simulink model "CPS_PowerSync_System"  (R2024a)
settings: Solver=FixedStepAuto  StartTime=0.0  StopTime=50  FixedStep=0.1  RelTol=1e-3
model workspace (MAT data in the model file):
  SoC = Simulink.Signal
  SoC.DataType = 'double'
  SoC.Dimensions = -1
  SoC.DimensionsMode = 'auto'
  SoC.Complexity = 'auto'
  SoC.SampleTime = -1
  SoC.SamplingMode = 'auto'
undefined symbols (not defined in the file or in its folder): m, v_CP1, v_CP2, v_CP3, w_CP1, w_CP2, w_CP3
(part 1 of 3)
settings Model: SimulationMode=accelerator  SnapshotBufferSize=100  SnapshotInterval=1  Creator=rober  LastModifiedBy=gabri
settings SolverCC: ConcurrentTasks=on  AutoInsertRateTranBlk=on
settings DebuggingCC: BusObjectLabelMismatch=none  UnderSpecifiedDimensionMsg=warning

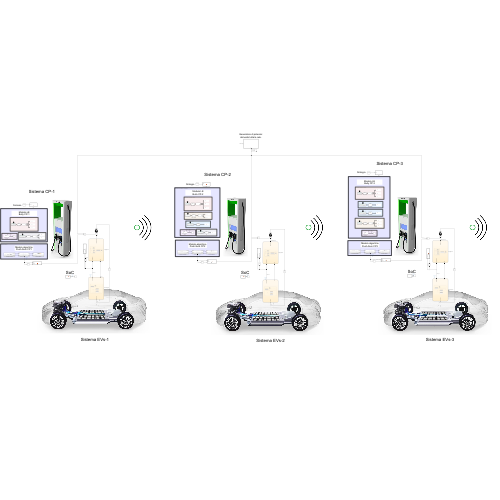
[thumbnail: Simulink's stored preview of the top-level diagram]
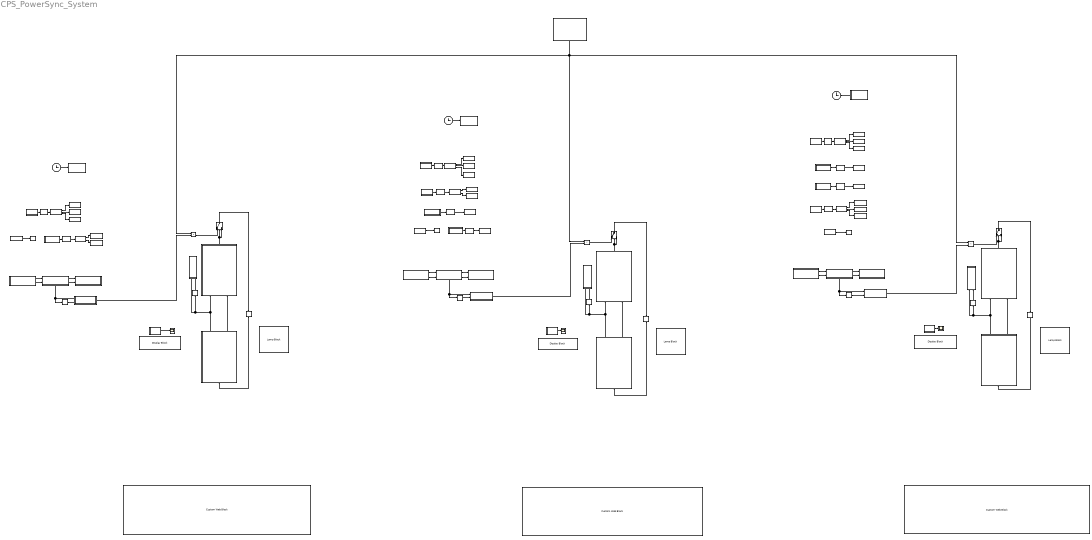
== system CPS_PowerSync_System ==
  note: Sistema EVs-3
  note: Answer module for LE
  note: Send Module
  note: Receive module
  note: Charging point 1 | UID 1 | LE module 1
  note: Charging Point 3 | UID 3 | LE module 3
  note: Charging point 2 | UID 2 | LE module 2
  note: Receive module
  note: Send Module
  note: Receive module
  note: Leader dead notification module
  note: Push-sum module 3
  note: Push-sum module 1
  note: Push-sum module 2
  note: Orologio
  note: Modulo LE
      | Bully CP-1
  note: Modulo algoritmo
      | Push-Sum CP1
  note: Modulo algoritmo
      | Push-Sum CP2
  note: Modulo algoritmo
      | Push-Sum CP3
  note: Answer module for LE
  note: Election notification module
  note: Generatore di potenza: alimenta tutta la rete.
  note: Sistema CP-2
  note: Sistema CP-3
  note: Sistema CP-1
  note: Sistema EVs-1
  note: Sistema EVs-2
  note: SoC
  note: Modulo LE
      | Bully CP-2
  note: Modulo LE
      | Bully CP-3
  note: Leader dead notification module
  note: Election notification module
  note: Orologio
  note: Orologio
  note: Leader dead notification module
  note: Answer module for LE
  note: SoC
  note: SoC
  CP 1 : EntityGenerator  InputPortMessageModes=m  OutputPortMessageModes=m  GenerationMethod=Event-based  TimeSource=Signal port  Period=3  AttributeName=UID  EntityType=Structured  EntityTypeName=Entity
      settings: InputPortMap=u0
  CP 2 : EntityGenerator  InputPortMessageModes=m  OutputPortMessageModes=m  GenerationMethod=Event-based  TimeSource=Signal port  Period=3  AttributeName=UID  AttributeInitialValue=2  EntityType=Structured  EntityTypeName=Entity
      settings: InputPortMap=u0
  CP1 : MATLAB Function  TreatAsAtomicUnit=on
  CP2 : MATLAB Function  TreatAsAtomicUnit=on
  CP3 : MATLAB Function  TreatAsAtomicUnit=on
  ChargingPoint1 : Stateflow chart  TreatAsAtomicUnit=on
  ChargingPoint2 : Stateflow chart  TreatAsAtomicUnit=on
  ChargingPoint3 : Stateflow chart  TreatAsAtomicUnit=on
  Clock1 : Clock
  Clock2 : Clock
  Clock3 : Clock
  Delay{,1..8} (9 alike) : Delay  DelayLength=1  InitialCondition=0  SampleTime=0.1
  Display : DisplayBlock  LabelPosition=Hide  Transparency=1
  Display2 : DisplayBlock  LabelPosition=Hide  Transparency=1
  Display3 : DisplayBlock  LabelPosition=Hide  Transparency=1
  ElecritcVehicles1 : Stateflow chart  TreatAsAtomicUnit=on
  ElecritcVehicles2 : Stateflow chart  TreatAsAtomicUnit=on
  ElecritcVehicles3 : Stateflow chart  TreatAsAtomicUnit=on
  Entity Multicast{,6,8,11,13..14,16} (7 alike) : EntityMulticast  Tag=B  InputPortMessageModes=m  MulticastTag=B
  Entity Multicast{1,4,7,9..10,18..19} (7 alike) : EntityMulticast  Tag=A  InputPortMessageModes=m
  Entity Multicast{2..3,5,12,15,17} (6 alike) : EntityMulticast  Tag=C  InputPortMessageModes=m  MulticastTag=C
  Entity Replicator{,1,4..5} (4 alike) : EntityReplicator  InputPortMessageModes=m  OutputPortMessageModes=m,m,m  NumberReplicas=2
      settings: OutputPortMap=o0,o1,o2
  Entity Replicator2 : EntityReplicator  InputPortMessageModes=m  OutputPortMessageModes=m,m
  Entity Replicator3 : EntityReplicator  InputPortMessageModes=m  OutputPortMessageModes=m,m
  Entity Terminator : EntityTerminator  InputPortMessageModes=m  EntryAction=|
      | coder.extrinsic('evalin');
      | coder.extrinsic('assignin');
      | 
      | check_variables('v_CP1');
      | 
      | clock = 0;
      | clock = evalin('base', 'clock_CP1');
      | 
      | pr_actual = 0;
      | pr_actual = evalin('base', 'double(pr_actual_CP1)');
      | 
      | if pr_actual == 0
      |     assignin('base', 'v_CP1', 0); % Non sono leader
      | end
      | 
      | % Caso in cui ricevo un UID maggiore del mio
      | if entity.UID > 1
      |     assignin('base', 'flg_response_CP1', 1);
      |     assignin('base', 'v_CP1', 0); % Non sono leader
      |     disp('CP1 received a UID greater than its own, so it knows that it will not be the leader.')
      | end
      | 
      | 
      | % Caso in cui ricevo messaggio di elezione avvenuta e sono connesso
      | if entity.UID == -2 && pr_actual == 1
      |     
      |     % Elezione avvenuta
      |     % Tutti e tre questi flag sono necessari al corretto funzionamento dell'algoritmo push-sum
      |     assignin('base', 'flg_elected_CP1', 1);
      |     assignin('base', 'flg_first_instant_v_CP1', 1);
      |     assignin('base', 'flg_first_instant_w_CP1', 1);
      | 
      |     assignin('base', 'flg_send_CP1', 0);
      |     
      |     disp('CP1 is active and has learned that the leader has been elected (received -2).')
      | 
      | end
      | 
      | 
      | % Ricevo notifica morte leader
      | if entity.UID == -1
      |     
      |     disp('CP1 heard that the leader died (received -1)')
      |     
      |     % Reset del valore e del peso
      |     assignin('base', 'v_CP1', 0);
      |     assignin('base', 'w_CP1', 0);
      |     
      |     % Il leader deve essere rieletto, quindi flag_elected viene riportato a zero
      |     assignin('base', 'flg_elected_CP1', 0);
      |     
      |     % Il nodo si propone come leader e, nel caso in cui riceverà
      |     % una risposta, questo flag sarà impostato = 1
      |     assignin('base', 'flg_response_CP1', 0);
      |     
      |     % Flag necessari a far ripartire l'algoritmo push-sum correttamente
      |     assignin('base', 'flg_dead_v_CP1', 1);
      |     assignin('base', 'flg_dead_w_CP1', 1);
      |     assignin('base', 'flg_reset_v_CP1', 1);
      |     assignin('base', 'flg_reset_w_CP1', 1);
      | 
      |     if pr_actual == 1
      |         
      |         disp('CP1 sent its candidacy.')
      | 
      |         % Il nodo si propone come leader inviando il messaggio
      |         get_event_CP1();
      |         assignin('base', 'flg_send_CP1', 1);
      |         
      |         % Stacco il tempo (tempo di invio del messaggio)
      |         assignin('base', 't_send_CP1', clock);
      |         
      |     end
      | 
      | end
  Entity Terminator1 : EntityTerminator  InputPortMessageModes=m  EntryAction=|
      | coder.extrinsic('evalin');
      | coder.extrinsic('assignin');
      | 
      | check_variables('v_CP2');
      | 
      | clock = 0;
      | clock = evalin('base', 'clock_CP2');
      | 
      | pr_actual = 0;
      | pr_actual = evalin('base', 'double(pr_actual_CP2)');
      | 
      | t_send = 0;
      | t_send = evalin('base', 't_send_CP2');
      | 
      | if pr_actual == 0
      |     assignin('base', 'v_CP2', 0); % Non sono leader
      | end
      | 
      | 
      | % Caso in cui ricevo un UID maggiore del mio
      | if entity.UID > 2
      |     assignin('base', 'flg_response_CP2', 1);
      |     assignin('base', 'v_CP2', 0); % Non sono leader
      |     disp('CP2 received a UID greater than its own, so it knows that it will not be the leader.')
      | end
      | 
      | 
      | % Se sei connesso e ti contatta un nodo con UID più piccolo rispondi
      | if entity.UID < 2 && entity.UID > 0 && pr_actual == 1
      |     
      |     response_2_to_1();
      |     
      |     assignin('base', 'flg_send_CP2', 1);
      |     
      |     if (clock - t_send) > 1
      |         assignin('base', 't_send_CP2', clock);
      |     end
      |     
      |     disp('CP2 received UID = 1, so it responds to CP1.')
      |     
      | end
      | 
      | % Caso in cui ricevo messaggio di elezione avvenuta e sono connesso
      | if entity.UID == -2 && pr_actual == 1
      |     
      |     % Elezione avvenuta
      |     % Tutti e tre questi flag sono necessari al corretto funzionamento dell'algoritmo push-sum
      |     assignin('base', 'flg_elected_CP2', 1);
      |     assignin('base', 'flg_first_instant_v_CP2', 1);
      |     assignin('base', 'flg_first_instant_w_CP2', 1);
      | 
      |     assignin('base', 'flg_send_CP2', 0);
      |     
      |     disp('CP2 is active and has learned that the leader has been elected (received -2).')
      | 
      | end
      | 
      | 
      | % Ricevo notifica morte leader
      | if entity.UID == -1
      |     
      |     disp('CP2 heard that the leader died (received -1)')
      |     
      |     % Reset del valore e del peso
      |     assignin('base', 'v_CP2', 0);
      |     assignin('base', 'w_CP2', 0);
      |     
      |     % Il leader deve essere rieletto, quindi flag_elected viene riportato a zero
      |     assignin('base', 'flg_elected_CP2', 0);
      |     
      |     % Il nodo si propone come leader e, nel caso in cui riceverà
      |     % una risposta, questo flag sarà impostato = 1
      |     assignin('base', 'flg_response_CP2', 0);
      |     
      |     % Flag necessari a far ripartire l'algoritmo push-sum correttamente
      |     assignin('base', 'flg_dead_v_CP2', 1);
      |     assignin('base', 'flg_dead_w_CP2', 1);
      |     assignin('base', 'flg_reset_v_CP2', 1);
      |     assignin('base', 'flg_reset_w_CP2', 1);
      | 
      |     if pr_actual == 1
      |         
      |         disp('CP2 sent its candidacy.')
      | 
      |         % Il nodo si propone come leader inviando il messaggio
      |         get_event_CP2();
      |         assignin('base', 'flg_send_CP2', 1);
      |         
      |         % Stacco il tempo (tempo di invio del messaggio)
      |         assignin('base', 't_send_CP2', clock);
      |         
      |     end
      | 
      | end
  Entity Terminator2 : EntityTerminator  InputPortMessageModes=m  EntryAction=|
      | coder.extrinsic('evalin');
      | coder.extrinsic('assignin');
      | 
      | check_variables('v_CP3');
      | 
      | clock = 0;
      | clock = evalin('base', 'clock_CP3');
      | 
      | pr_actual = 0;
      | pr_actual = evalin('base', 'double(pr_actual_CP3)');
      | 
      | t_send = 0;
      | t_send = evalin('base', 't_send_CP3');
      | 
      | if pr_actual == 0
      |     assignin('base', 'v_CP3', 0); % Non sono leader
      | end
      | 
      | 
      | % Caso in cui ricevo un UID maggiore del mio
      | if entity.UID > 3
      |     assignin('base', 'flg_response_CP3', 1);
      |     assignin('base', 'v_CP3', 0); % Non sono leader
      |     disp('CP3 received a UID greater than its own, so it knows that it will not be the leader.')
      | end
      | 
      | 
      | % Se sei connesso e ti contatta un nodo con UID più piccolo rispondi
      | if entity.UID < 3 && entity.UID > 0 && pr_actual == 1
      |     
      |     assignin('base', 'flg_send_CP3', 1);
      |     
      |     if (clock - t_send) > 1
      |         assignin('base', 'clock_CP3', clock);
      |     end
      |     
      |     if entity.UID == 1
      |         response_3_to_1();
      |         disp('CP3 received UID = 1, so it responds to CP1.')  
      |     else
      |         response_3_to_2();
      |         disp('CP3 received UID = 2, so it responds to CP2.')
      |     end
      |     
      | end
      | 
      | % Caso in cui ricevo messaggio di elezione avvenuta e sono connesso
      | if entity.UID == -2 && pr_actual == 1
      |     
      |     % Elezione avvenuta
      |     % Tutti e tre questi flag sono necessari al corretto funzionamento dell'algoritmo push-sum
      |     assignin('base', 'flg_elected_CP3', 1);
      |     assignin('base', 'flg_first_instant_v_CP3', 1);
      |     assignin('base', 'flg_first_instant_w_CP3', 1);
      | 
      |     assignin('base', 'flg_send_CP3', 0);
      |     
      |     disp('CP3 is active and has learned that the leader has been elected (received -2).')
      | 
      | end
      | 
      | 
      | % Ricevo notifica morte leader
      | if entity.UID == -1
      |     
      |     disp('CP3 heard that the leader died (received -1)')
      |     
      |     % Reset del valore e del peso
      |     assignin('base', 'v_CP3', 0);
      |     assignin('base', 'w_CP3', 0);
      |     
      |     % Il leader deve essere rieletto, quindi flag_elected viene riportato a zero
      |     assignin('base', 'flg_elected_CP3', 0);
      |     
      |     % Il nodo si propone come leader e, nel caso in cui riceverà
      |     % una risposta, questo flag sarà impostato = 1
      |     assignin('base', 'flg_response_CP3', 0);
      |     
      |     % Flag necessari a far ripartire l'algoritmo push-sum correttamente
      |     assignin('base', 'flg_dead_v_CP3', 1);
      |     assignin('base', 'flg_dead_w_CP3', 1);
      |     assignin('base', 'flg_reset_v_CP3', 1);
      |     assignin('base', 'flg_reset_w_CP3', 1);
      | 
      |     if pr_actual == 1
      |         
      |         disp('CP3 sent its candidacy.')
      | 
      |         % Il nodo si propone come leader inviando il messaggio
      |         assignin('base', 'flg_send_CP3', 1);
      |         
      |         % Stacco il tempo (tempo di invio del messaggio)
      |         assignin('base', 't_send_CP3', clock);
      |         
      |     end
      | 
      | end
  Entity risposta : EntityGenerator  InputPortMessageModes=m  OutputPortMessageModes=m  GenerationMethod=Event-based  TimeSource=Signal port  Period=3  AttributeName=UID  AttributeInitialValue=999  EntityType=Structured  EntityTypeName=Entity
      settings: InputPortMap=u0
  Entity risposta1 : EntityGenerator  InputPortMessageModes=m  OutputPortMessageModes=m  GenerationMethod=Event-based  TimeSource=Signal port  Period=3  AttributeName=UID  AttributeInitialValue=999  EntityType=Structured  EntityTypeName=Entity
      settings: InputPortMap=u0
  Entity risposta2 : EntityGenerator  InputPortMessageModes=m  OutputPortMessageModes=m  GenerationMethod=Event-based  TimeSource=Signal port  Period=3  AttributeName=UID  AttributeInitialValue=-2  EntityType=Structured  EntityTypeName=Entity
      settings: InputPortMap=u0
  Entity risposta3 : EntityGenerator  InputPortMessageModes=m  OutputPortMessageModes=m  GenerationMethod=Event-based  TimeSource=Signal port  Period=3  AttributeName=UID  AttributeInitialValue=-2  EntityType=Structured  EntityTypeName=Entity
      settings: InputPortMap=u0
  Entity risposta4 : EntityGenerator  InputPortMessageModes=m  OutputPortMessageModes=m  GenerationMethod=Event-based  TimeSource=Signal port  Period=3  AttributeName=UID  AttributeInitialValue=-1  EntityType=Structured  EntityTypeName=Entity
      settings: InputPortMap=u0
  Entity risposta5 : EntityGenerator  InputPortMessageModes=m  OutputPortMessageModes=m  GenerationMethod=Event-based  TimeSource=Signal port  Period=3  AttributeName=UID  AttributeInitialValue=-1  EntityType=Structured  EntityTypeName=Entity
      settings: InputPortMap=u0
  Entity risposta6 : EntityGenerator  InputPortMessageModes=m  OutputPortMessageModes=m  GenerationMethod=Event-based  TimeSource=Signal port  Period=3  AttributeName=UID  AttributeInitialValue=-1  EntityType=Structured  EntityTypeName=Entity
      settings: InputPortMap=u0
  Entity risposta7 : EntityGenerator  InputPortMessageModes=m  OutputPortMessageModes=m  GenerationMethod=Event-based  TimeSource=Signal port  Period=3  AttributeName=UID  AttributeInitialValue=999  EntityType=Structured  EntityTypeName=Entity
      settings: InputPortMap=u0
  Horizontal Gauge : CustomWebBlock  LabelPosition=Hide  ShowInitialText=on  Configuration="{\"components\":[{\"name\":\"LinearScaleComponent\",\"settings\":{\"bounds\":{\"max\":1,\"min\":0,\"tickInterval\":0.2},\"internalTickHeightScaleFactor\":0.5,\"labelColor\":[255,255,200],\"labelFont\":{\"font\":\"Arial\",\"fontSize\":12},\"labelOffset\":0.05,\"labelTransparency\":1,\"needleImage\":{\"size\":[21,75],\"src\":\"data:image\\/svg+xml;base64,PHN2ZyB4bWxucz0iaHR0cDovL3d3dy53My5vcmcvMjAwMC9zdmciIHhtbG5zOnhsaW5rPSJodHRwOi8vd3d3LnczLm9yZy8xOTk5L3hsaW5rIiB2aWV3Qm94PSIwIDAgMjEgNzUiPjxkZWZzPjxzdHlsZT4uY2xzLTF7ZmlsbDpub25lO30uY2xzLTJ7aXNvbGF0aW9uOmlzb2xhdGU7fS5jbHMtM3tjbGlwLXBhdGg6dXJsKCNjbGlwLXBhdGgpO30uY2xzLTR7b3BhY2l0eTowLjM7bWl4LWJsZW5kLW1vZGU6bXVsdGlwbHk7fS5jbHMtNXtmaWxsOiNlYjI2Mjk7fTwvc3R5bGU+PGNsaXBQYXRoIGlkPSJjbGlwLXBhdGgiIHRyYW5zZm9y ...(+1928 chars)\",\"srcOrientation\":\"Right\"},\"needleOffset\":[0,-0.007413509060955519],\"needleSize\":{\"height\":0.7589285714285714,\"width\":0.11955094537815127},\"position\":[0.06969246031746032,0.01995798319327731,0.9641544117647058,0.7998511904761905],\"referencePoint\":\"auto\",\"scaleColors\":[],\"scaleColorsSize\":0.2,\"scaleDirection\":\"LR\",\"showLabels\":1,\"showMinorTicks\":0,\"showSpanLine\":1,\"showTicks\":1,\"tickColor\":[252,252,197],\"tickTransparency\":1,\"valueBarColor\":[23,89,176],\"valueBarOffset\":0,\"valueBarSize\":0.23,\"valueBarTransparency\":1}},{\"name\":\"BackgroundImageComponent\",\"settings\":{\"image\":{\"size\":[380,101],\"src\":\"data:image\\/svg+xml;base64,PHN2ZyBpZD0iZnJhbWUiIHhtbG5zPSJodHRwOi8vd3d3LnczLm9yZy8yMDAwL3N2ZyIgeG1sbnM6eGxpbms9Imh0dHA6Ly93d3cudzMub3JnLzE5OTkveGxpbmsiIHZpZXdCb3g9IjAgMCAzODAgMTAxIj48ZGVmcz48c3R5bGU+LmNscy0xe2ZpbGw6IzAwMmI0Mjt9LmNscy0ye2ZpbGw6IzQyNzA4Mjt9LmNscy0ze2ZpbGw6dXJsKCNyYWRpYWwtZ3JhZGllbnQpO308L3N0eWxlPjxyYWRpYWxHcmFkaWVudCBpZD0icmFkaWFsLWdyYWRpZW50IiBjeD0iMTkwIiBjeT0iNTAuNSIgcj0iMjY5LjIxIiBncmFkaWVudFVuaXRzPSJ1c2VyU3BhY2VPblVzZSI+PHN0b3Agb2Zmc2V0PSIwLjAxIiBzdG9wLWNvbG9yPSIjM2U0ZjU4Ii8+PHN0b3Agb2Zmc2V0PSIwLjA2IiBzdG9wLWNvbG9yPSIjNDQ1NzYxIi8+PHN0b3Agb2Zmc2V0PSIwLjE1IiBzdG9wLWNvbG9yPSIjNTU2YTc2Ii8+PHN0b3Agb2Zmc2V0PSIwLjI1IiBzdG9wLWNvbG9yPSIjNmQ4ODk1Ii8+PHN0b3Agb2Zmc2V0PSIwLjM4IiBzdG9wLWNvbG9yPSIjOGZiMmMzIi8+PHN0b3Agb2Zmc2V0PSIwLjUyIiBzdG9wLWNvbG9yPSIjYjZlNGZhIi8+PHN0b3Agb2Zmc2V0PSIxIiBzdG9wLWNvbG9yPSIjMTU0NjU3Ii8+PC9yYWRpYWxHcmFkaWVudD48L2RlZnM+PGcgaWQ9IkxheWVyXzIiIGRhdGEtbmFtZT0iTGF5ZXIgMiI+PGcgaWQ9IkxheWVyXzEtMiIgZGF0YS1uYW1lPSJMYXllciAxLTIiPjxyZWN0IGlkPSJyZWN0MTAzNiIgY2xhc3M9ImNscy0xIiB4PSIxMSIgeT0iMTEiIHdpZHRoPSIzNTgiIGhlaWdodD0iNzkiLz48cGF0aCBpZD0icGF0aDEwMzgiIGNsYXNzPSJjbHMtMiIgZD0iTTgsOFY5M0gzNzJWOFpNMzY5LDkwSDExVjExSDM2OVoiLz48cGF0aCBpZD0icGF0aDEwNDAiIGNsYXNzPSJjbHMtMyIgZD0iTTAsMFYxMDFIMzgwVjBaTTM3Miw5M0g4VjhIMzcyWiIvPjwvZz48L2c+PC9zdmc+\",\"srcOrientation\":\"horizontal\"},\"position\":[0,0,1,1],\"scaleMode\":\"0\"}},{\"name\":\"ForegroundImageComponent\",\"settings\":{\"image\":{\"size\":[0,0],\"src\":\"default\",\"srcOrientation\":[]},\"isForeground\":1,\"position\":[0,0,1,1],\"scaleMode\":\"0\"}}],\"settings\":{\"BindingType\":\"signal\",\"backgroundColor\":[0,0,0,\"1\"],\"backgroundOffset\":0,\"backgroundOpacity\":1,\"fixedAspectRatio\":\"on\",\"orientation\":\"horizontal\",\"showBackgroundColor\":false,\"value\":0,\"version\":\"R2023a\"},\"type\":\"LinearGauge\"}"
  Horizontal Gauge1 : CustomWebBlock  LabelPosition=Hide  ShowInitialText=on  Configuration="{\"components\":[{\"name\":\"LinearScaleComponent\",\"settings\":{\"bounds\":{\"max\":1,\"min\":0,\"tickInterval\":0.2},\"internalTickHeightScaleFactor\":0.5,\"labelColor\":[255,255,200],\"labelFont\":{\"font\":\"Arial\",\"fontSize\":12},\"labelOffset\":0.05,\"labelTransparency\":1,\"needleImage\":{\"size\":[21,75],\"src\":\"data:image\\/svg+xml;base64,PHN2ZyB4bWxucz0iaHR0cDovL3d3dy53My5vcmcvMjAwMC9zdmciIHhtbG5zOnhsaW5rPSJodHRwOi8vd3d3LnczLm9yZy8xOTk5L3hsaW5rIiB2aWV3Qm94PSIwIDAgMjEgNzUiPjxkZWZzPjxzdHlsZT4uY2xzLTF7ZmlsbDpub25lO30uY2xzLTJ7aXNvbGF0aW9uOmlzb2xhdGU7fS5jbHMtM3tjbGlwLXBhdGg6dXJsKCNjbGlwLXBhdGgpO30uY2xzLTR7b3BhY2l0eTowLjM7bWl4LWJsZW5kLW1vZGU6bXVsdGlwbHk7fS5jbHMtNXtmaWxsOiNlYjI2Mjk7fTwvc3R5bGU+PGNsaXBQYXRoIGlkPSJjbGlwLXBhdGgiIHRyYW5zZm9y ...(+1928 chars)\",\"srcOrientation\":\"Right\"},\"needleOffset\":[0,-0.007413509060955519],\"needleSize\":{\"height\":0.7589285714285714,\"width\":0.11955094537815127},\"position\":[0.06969246031746032,0.01995798319327731,0.9641544117647058,0.7998511904761905],\"referencePoint\":\"auto\",\"scaleColors\":[],\"scaleColorsSize\":0.2,\"scaleDirection\":\"LR\",\"showLabels\":1,\"showMinorTicks\":0,\"showSpanLine\":1,\"showTicks\":1,\"tickColor\":[252,252,197],\"tickTransparency\":1,\"valueBarColor\":[23,89,176],\"valueBarOffset\":0,\"valueBarSize\":0.23,\"valueBarTransparency\":1}},{\"name\":\"BackgroundImageComponent\",\"settings\":{\"image\":{\"size\":[380,101],\"src\":\"data:image\\/svg+xml;base64,PHN2ZyBpZD0iZnJhbWUiIHhtbG5zPSJodHRwOi8vd3d3LnczLm9yZy8yMDAwL3N2ZyIgeG1sbnM6eGxpbms9Imh0dHA6Ly93d3cudzMub3JnLzE5OTkveGxpbmsiIHZpZXdCb3g9IjAgMCAzODAgMTAxIj48ZGVmcz48c3R5bGU+LmNscy0xe2ZpbGw6IzAwMmI0Mjt9LmNscy0ye2ZpbGw6IzQyNzA4Mjt9LmNscy0ze2ZpbGw6dXJsKCNyYWRpYWwtZ3JhZGllbnQpO308L3N0eWxlPjxyYWRpYWxHcmFkaWVudCBpZD0icmFkaWFsLWdyYWRpZW50IiBjeD0iMTkwIiBjeT0iNTAuNSIgcj0iMjY5LjIxIiBncmFkaWVudFVuaXRzPSJ1c2VyU3BhY2VPblVzZSI+PHN0b3Agb2Zmc2V0PSIwLjAxIiBzdG9wLWNvbG9yPSIjM2U0ZjU4Ii8+PHN0b3Agb2Zmc2V0PSIwLjA2IiBzdG9wLWNvbG9yPSIjNDQ1NzYxIi8+PHN0b3Agb2Zmc2V0PSIwLjE1IiBzdG9wLWNvbG9yPSIjNTU2YTc2Ii8+PHN0b3Agb2Zmc2V0PSIwLjI1IiBzdG9wLWNvbG9yPSIjNmQ4ODk1Ii8+PHN0b3Agb2Zmc2V0PSIwLjM4IiBzdG9wLWNvbG9yPSIjOGZiMmMzIi8+PHN0b3Agb2Zmc2V0PSIwLjUyIiBzdG9wLWNvbG9yPSIjYjZlNGZhIi8+PHN0b3Agb2Zmc2V0PSIxIiBzdG9wLWNvbG9yPSIjMTU0NjU3Ii8+PC9yYWRpYWxHcmFkaWVudD48L2RlZnM+PGcgaWQ9IkxheWVyXzIiIGRhdGEtbmFtZT0iTGF5ZXIgMiI+PGcgaWQ9IkxheWVyXzEtMiIgZGF0YS1uYW1lPSJMYXllciAxLTIiPjxyZWN0IGlkPSJyZWN0MTAzNiIgY2xhc3M9ImNscy0xIiB4PSIxMSIgeT0iMTEiIHdpZHRoPSIzNTgiIGhlaWdodD0iNzkiLz48cGF0aCBpZD0icGF0aDEwMzgiIGNsYXNzPSJjbHMtMiIgZD0iTTgsOFY5M0gzNzJWOFpNMzY5LDkwSDExVjExSDM2OVoiLz48cGF0aCBpZD0icGF0aDEwNDAiIGNsYXNzPSJjbHMtMyIgZD0iTTAsMFYxMDFIMzgwVjBaTTM3Miw5M0g4VjhIMzcyWiIvPjwvZz48L2c+PC9zdmc+\",\"srcOrientation\":\"horizontal\"},\"position\":[0,0,1,1],\"scaleMode\":\"0\"}},{\"name\":\"ForegroundImageComponent\",\"settings\":{\"image\":{\"size\":[0,0],\"src\":\"default\",\"srcOrientation\":[]},\"isForeground\":1,\"position\":[0,0,1,1],\"scaleMode\":\"0\"}}],\"settings\":{\"BindingType\":\"signal\",\"backgroundColor\":[0,0,0,\"1\"],\"backgroundOffset\":0,\"backgroundOpacity\":1,\"fixedAspectRatio\":\"on\",\"orientation\":\"horizontal\",\"showBackgroundColor\":false,\"value\":0,\"version\":\"R2023a\"},\"type\":\"LinearGauge\"}"
  Horizontal Gauge2 : CustomWebBlock  LabelPosition=Hide  ShowInitialText=on  Configuration="{\"components\":[{\"name\":\"LinearScaleComponent\",\"settings\":{\"bounds\":{\"max\":1,\"min\":0,\"tickInterval\":0.2},\"internalTickHeightScaleFactor\":0.5,\"labelColor\":[255,255,200],\"labelFont\":{\"font\":\"Arial\",\"fontSize\":12},\"labelOffset\":0.05,\"labelTransparency\":1,\"needleImage\":{\"size\":[21,75],\"src\":\"data:image\\/svg+xml;base64,PHN2ZyB4bWxucz0iaHR0cDovL3d3dy53My5vcmcvMjAwMC9zdmciIHhtbG5zOnhsaW5rPSJodHRwOi8vd3d3LnczLm9yZy8xOTk5L3hsaW5rIiB2aWV3Qm94PSIwIDAgMjEgNzUiPjxkZWZzPjxzdHlsZT4uY2xzLTF7ZmlsbDpub25lO30uY2xzLTJ7aXNvbGF0aW9uOmlzb2xhdGU7fS5jbHMtM3tjbGlwLXBhdGg6dXJsKCNjbGlwLXBhdGgpO30uY2xzLTR7b3BhY2l0eTowLjM7bWl4LWJsZW5kLW1vZGU6bXVsdGlwbHk7fS5jbHMtNXtmaWxsOiNlYjI2Mjk7fTwvc3R5bGU+PGNsaXBQYXRoIGlkPSJjbGlwLXBhdGgiIHRyYW5zZm9y ...(+1928 chars)\",\"srcOrientation\":\"Right\"},\"needleOffset\":[0,-0.007413509060955519],\"needleSize\":{\"height\":0.7589285714285714,\"width\":0.11955094537815127},\"position\":[0.06969246031746032,0.01995798319327731,0.9641544117647058,0.7998511904761905],\"referencePoint\":\"auto\",\"scaleColors\":[],\"scaleColorsSize\":0.2,\"scaleDirection\":\"LR\",\"showLabels\":1,\"showMinorTicks\":0,\"showSpanLine\":1,\"showTicks\":1,\"tickColor\":[252,252,197],\"tickTransparency\":1,\"valueBarColor\":[23,89,176],\"valueBarOffset\":0,\"valueBarSize\":0.23,\"valueBarTransparency\":1}},{\"name\":\"BackgroundImageComponent\",\"settings\":{\"image\":{\"size\":[380,101],\"src\":\"data:image\\/svg+xml;base64,PHN2ZyBpZD0iZnJhbWUiIHhtbG5zPSJodHRwOi8vd3d3LnczLm9yZy8yMDAwL3N2ZyIgeG1sbnM6eGxpbms9Imh0dHA6Ly93d3cudzMub3JnLzE5OTkveGxpbmsiIHZpZXdCb3g9IjAgMCAzODAgMTAxIj48ZGVmcz48c3R5bGU+LmNscy0xe2ZpbGw6IzAwMmI0Mjt9LmNscy0ye2ZpbGw6IzQyNzA4Mjt9LmNscy0ze2ZpbGw6dXJsKCNyYWRpYWwtZ3JhZGllbnQpO308L3N0eWxlPjxyYWRpYWxHcmFkaWVudCBpZD0icmFkaWFsLWdyYWRpZW50IiBjeD0iMTkwIiBjeT0iNTAuNSIgcj0iMjY5LjIxIiBncmFkaWVudFVuaXRzPSJ1c2VyU3BhY2VPblVzZSI+PHN0b3Agb2Zmc2V0PSIwLjAxIiBzdG9wLWNvbG9yPSIjM2U0ZjU4Ii8+PHN0b3Agb2Zmc2V0PSIwLjA2IiBzdG9wLWNvbG9yPSIjNDQ1NzYxIi8+PHN0b3Agb2Zmc2V0PSIwLjE1IiBzdG9wLWNvbG9yPSIjNTU2YTc2Ii8+PHN0b3Agb2Zmc2V0PSIwLjI1IiBzdG9wLWNvbG9yPSIjNmQ4ODk1Ii8+PHN0b3Agb2Zmc2V0PSIwLjM4IiBzdG9wLWNvbG9yPSIjOGZiMmMzIi8+PHN0b3Agb2Zmc2V0PSIwLjUyIiBzdG9wLWNvbG9yPSIjYjZlNGZhIi8+PHN0b3Agb2Zmc2V0PSIxIiBzdG9wLWNvbG9yPSIjMTU0NjU3Ii8+PC9yYWRpYWxHcmFkaWVudD48L2RlZnM+PGcgaWQ9IkxheWVyXzIiIGRhdGEtbmFtZT0iTGF5ZXIgMiI+PGcgaWQ9IkxheWVyXzEtMiIgZGF0YS1uYW1lPSJMYXllciAxLTIiPjxyZWN0IGlkPSJyZWN0MTAzNiIgY2xhc3M9ImNscy0xIiB4PSIxMSIgeT0iMTEiIHdpZHRoPSIzNTgiIGhlaWdodD0iNzkiLz48cGF0aCBpZD0icGF0aDEwMzgiIGNsYXNzPSJjbHMtMiIgZD0iTTgsOFY5M0gzNzJWOFpNMzY5LDkwSDExVjExSDM2OVoiLz48cGF0aCBpZD0icGF0aDEwNDAiIGNsYXNzPSJjbHMtMyIgZD0iTTAsMFYxMDFIMzgwVjBaTTM3Miw5M0g4VjhIMzcyWiIvPjwvZz48L2c+PC9zdmc+\",\"srcOrientation\":\"horizontal\"},\"position\":[0,0,1,1],\"scaleMode\":\"0\"}},{\"name\":\"ForegroundImageComponent\",\"settings\":{\"image\":{\"size\":[0,0],\"src\":\"default\",\"srcOrientation\":[]},\"isForeground\":1,\"position\":[0,0,1,1],\"scaleMode\":\"0\"}}],\"settings\":{\"BindingType\":\"signal\",\"backgroundColor\":[0,0,0,\"1\"],\"backgroundOffset\":0,\"backgroundOpacity\":1,\"fixedAspectRatio\":\"on\",\"orientation\":\"horizontal\",\"showBackgroundColor\":false,\"value\":0,\"version\":\"R2023a\"},\"type\":\"LinearGauge\"}"
  Lamp : LampBlock  LabelPosition=Hide
  Lamp1 : LampBlock  LabelPosition=Hide
  Lamp2 : LampBlock  LabelPosition=Hide
  MATLAB Function : MATLAB Function  TreatAsAtomicUnit=on
  MATLAB Function1 : MATLAB Function  TreatAsAtomicUnit=on
  MATLAB Function10 : MATLAB Function  TreatAsAtomicUnit=on
  MATLAB Function11 : MATLAB Function  TreatAsAtomicUnit=on
  MATLAB Function2 : MATLAB Function  TreatAsAtomicUnit=on
  MATLAB Function4 : MATLAB Function  TreatAsAtomicUnit=on
  MATLAB Function7 : MATLAB Function  TreatAsAtomicUnit=on
  MATLAB Function8 : MATLAB Function  TreatAsAtomicUnit=on
  MATLAB Function9 : MATLAB Function  TreatAsAtomicUnit=on
  Multicast Receive Queue : Queue  OutputPortMessageModes=m  EntityArrivalSource=Multicast  MulticastTag=B
  Multicast Receive Queue1 : Queue  OutputPortMessageModes=m  EntityArrivalSource=Multicast  MulticastTag=C
  Multicast Receive Queue2 : Queue  OutputPortMessageModes=m  EntityArrivalSource=Multicast
  Power supply : MATLAB Function  TreatAsAtomicUnit=on
  Product : Product
  Product1 : Product
  Product2 : Product
  Scope : Scope
  Scope1 : Scope
  Scope2 : Scope
  Simulink Function : Subsystem  TreatAsAtomicUnit=on
  Simulink Function1 : Subsystem  TreatAsAtomicUnit=on
  Simulink Function2 : Subsystem  TreatAsAtomicUnit=on
  Simulink Function3 : Subsystem  TreatAsAtomicUnit=on
  Simulink Function4 : Subsystem  TreatAsAtomicUnit=on
  Simulink Function5 : Subsystem  TreatAsAtomicUnit=on
  Simulink Function6 : Subsystem  TreatAsAtomicUnit=on
  Simulink Function7 : Subsystem  TreatAsAtomicUnit=on
  Simulink Function8 : Subsystem  TreatAsAtomicUnit=on
  Simulink Function9 : Subsystem  TreatAsAtomicUnit=on
  Subsystem : Subsystem
      settings: PortSchema="{\"entries\":[{\"content\":{\"sides\":[{\"content\":{\"connectorIds\":[\"In1\",\"In2\"]},\"type\":\"ConnectorPlacement.EquallySpacedRectSide\",\"uuid\":\"7bee7bec-1289-45e6-895e-15872bbdcddd\"},{\"content\":{\"connectorIds\":[\"Out1\",\"Out2\"],\"side\":\"RIGHT\"},\"type\":\"ConnectorPlacement.EquallySpacedRectSide\",\"uuid\":\"0edc84b3-335d-49a3-9bac-eca6380d867c\"},{\"content\":{\"side\":\"TOP\"},\"type\":\"ConnectorPlacement.EquallySpacedRectSide\",\"uuid\":\"45b2941a-719a-4af0-89a0-35288145da99\"},{\"content\":{\"connectorIds\":[\"Out3\"],\"side\":\"BOTTOM\"},\"type\":\"ConnectorPlacement.EquallySpacedRectSide\",\"uuid\":\"0edbb422-fd4b-4fbc-8ff5-1d5e9992019b\"}]},\"type\":\"ConnectorPlacement.EquallySpacedConnector\",\"uuid\":\"4d253b6f-5621-4e96-ac7d-189ebd944282\"}],\"packageUris\":[\"http://schema.mathworks.com/mf0/Connector/R2020b\"],\"version\":\"1.0\"}"
  Subsystem1 : Subsystem
      settings: PortSchema="{\"entries\":[{\"content\":{\"sides\":[{\"content\":{\"connectorIds\":[\"In1\",\"In2\"]},\"type\":\"ConnectorPlacement.EquallySpacedRectSide\",\"uuid\":\"7bee7bec-1289-45e6-895e-15872bbdcddd\"},{\"content\":{\"connectorIds\":[\"Out1\",\"Out2\"],\"side\":\"RIGHT\"},\"type\":\"ConnectorPlacement.EquallySpacedRectSide\",\"uuid\":\"0edc84b3-335d-49a3-9bac-eca6380d867c\"},{\"content\":{\"side\":\"TOP\"},\"type\":\"ConnectorPlacement.EquallySpacedRectSide\",\"uuid\":\"45b2941a-719a-4af0-89a0-35288145da99\"},{\"content\":{\"connectorIds\":[\"Out3\"],\"side\":\"BOTTOM\"},\"type\":\"ConnectorPlacement.EquallySpacedRectSide\",\"uuid\":\"0edbb422-fd4b-4fbc-8ff5-1d5e9992019b\"}]},\"type\":\"ConnectorPlacement.EquallySpacedConnector\",\"uuid\":\"4d253b6f-5621-4e96-ac7d-189ebd944282\"}],\"packageUris\":[\"http://schema.mathworks.com/mf0/Connector/R2020b\"],\"version\":\"1.0\"}"
  Subsystem2 : Subsystem
      settings: PortSchema="{\"entries\":[{\"content\":{\"sides\":[{\"content\":{\"connectorIds\":[\"In1\",\"In2\"]},\"type\":\"ConnectorPlacement.EquallySpacedRectSide\",\"uuid\":\"7bee7bec-1289-45e6-895e-15872bbdcddd\"},{\"content\":{\"connectorIds\":[\"Out1\",\"Out2\"],\"side\":\"RIGHT\"},\"type\":\"ConnectorPlacement.EquallySpacedRectSide\",\"uuid\":\"0edc84b3-335d-49a3-9bac-eca6380d867c\"},{\"content\":{\"side\":\"TOP\"},\"type\":\"ConnectorPlacement.EquallySpacedRectSide\",\"uuid\":\"45b2941a-719a-4af0-89a0-35288145da99\"},{\"content\":{\"connectorIds\":[\"Out3\"],\"side\":\"BOTTOM\"},\"type\":\"ConnectorPlacement.EquallySpacedRectSide\",\"uuid\":\"0edbb422-fd4b-4fbc-8ff5-1d5e9992019b\"}]},\"type\":\"ConnectorPlacement.EquallySpacedConnector\",\"uuid\":\"4d253b6f-5621-4e96-ac7d-189ebd944282\"}],\"packageUris\":[\"http://schema.mathworks.com/mf0/Connector/R2020b\"],\"version\":\"1.0\"}"
  Switch : Switch  Criteria=u2 > Threshold  SaturateOnIntegerOverflow=off  InputSameDT=off
  Switch1 : Switch  Criteria=u2 > Threshold  SaturateOnIntegerOverflow=off  InputSameDT=off
  Switch2 : Switch  Criteria=u2 > Threshold  SaturateOnIntegerOverflow=off  InputSameDT=off
  WirelessReceiveModule : Subsystem  SystemSampleTime=1
  WirelessReceiveModule1 : Subsystem
  WirelessReceiveModule2 : Subsystem
  WirelessSendModule : Subsystem
  WirelessSendModule1 : Subsystem
  WirelessSendModule2 : Subsystem
  wires:
  Simulink Function1/1(Out1) -> CP 2/1
  Multicast Receive Queue/1 -> Entity Terminator1/1
  Multicast Receive Queue1/1 -> Entity Terminator2/1
  CP 2/1 -> Entity Multicast3/1
  Simulink Function3/1(Out1) -> Entity risposta/1
  Entity risposta/1 -> Entity Multicast1/1
  Simulink Function4/1(Out1) -> Entity risposta1/1
  Entity risposta1/1 -> Entity Multicast6/1
  Entity Replicator2/1 -> Entity Multicast/1
  Simulink Function/1(Out1) -> CP 1/1
  Multicast Receive Queue2/1 -> Entity Terminator/1
  Entity Replicator2/2 -> Entity Multicast5/1
  CP 1/1 -> Entity Replicator2/1
  Simulink Function5/1(Out1) -> Entity risposta2/1
  Entity Replicator/1 -> Entity Multicast7/1
  Entity Replicator/2 -> Entity Multicast8/1
  Simulink Function7/1(Out1) -> Entity risposta4/1
  Entity Replicator1/1 -> Entity Multicast10/1
  Entity Replicator1/2 -> Entity Multicast11/1
  Entity Replicator1/3 -> Entity Multicast12/1
  WirelessReceiveModule2/1(<w2/2>) -> Subsystem2/1(w3/2)
  Subsystem1/2(w_CP2) -> WirelessSendModule1/2(w2/2)  "w2/2"
  Subsystem1/1(v_CP2) -> WirelessSendModule1/1(v2/2)  "v2/2"
  WirelessReceiveModule1/1(<w1/2>) -> Subsystem1/1(w_CP1)
  WirelessReceiveModule1/2(<v1/2>) -> Subsystem1/2(v_CP1)
  WirelessReceiveModule2/2(<v2/2>) -> Subsystem2/2(v3/2)
  Subsystem2/1(v2/2) -> WirelessSendModule2/1(v3/2)
  Subsystem2/2(w2/2) -> WirelessSendModule2/2(w3/2)
  Subsystem/1(v1/2) -> WirelessSendModule/1(v1/2)
  Subsystem/2(w1/2) -> WirelessSendModule/2(w1/2)
  WirelessReceiveModule/2(<v3/2>) -> Subsystem/2(v3/2)
  WirelessReceiveModule/1(<w3/2>) -> Subsystem/1(w3/2)
  Entity risposta2/1 -> Entity Replicator/1
  Entity Replicator/3 -> Entity Multicast2/1
  Subsystem1/3(Out2) -> Delay3/1, MATLAB Function8/1(actual)  "pushSum_CP2"
  Subsystem2/3(Out2) -> Delay7/1, MATLAB Function4/1(actual)  "pushSum_CP3"
  Subsystem/3(Out2) -> MATLAB Function7/1(actual), Delay/1  "pushSum_CP1"
  Delay5/1 -> ElecritcVehicles1/1(powerFlow)
  ChargingPoint1/1(enablePowerFlow) -> Switch/2, Switch/3
  ElecritcVehicles1/2(plug) -> ChargingPoint1/2(plug)  "plug_t1_1"
  ElecritcVehicles1/1(powerRequest) -> MATLAB Function10/1(pr_actual_CP1), Delay1/1, ChargingPoint1/1(powerRequest)  "pReq_CP1"
  Product/1 -> Switch/1
  Switch/1 -> Delay5/1
  MATLAB Function7/1(y) -> Product/2
  Delay/1 -> MATLAB Function7/2(previous)
  ChargingPoint2/1(enablePowerFlow) -> Switch1/2, Switch1/3
  Product1/1 -> Switch1/1
  Switch1/1 -> Delay4/1
  ElecritcVehicles2/2(plug) -> ChargingPoint2/2(plug)
  ElecritcVehicles2/1(powerRequest) -> ChargingPoint2/1(powerRequest), Delay2/1, MATLAB Function9/1(pr_actual_CP2)  "pReq_CP2"
  Delay4/1 -> ElecritcVehicles2/1(powerFlow)
  Delay2/1 -> MATLAB Function9/2(pr_previous_CP2)
  Delay3/1 -> MATLAB Function8/2(previous)
  MATLAB Function8/1(y) -> Product1/2
  Delay1/1 -> MATLAB Function10/2(pr_previous_CP1)  "plug_t0_1"
  ElecritcVehicles3/1(powerRequest) -> Delay6/1, MATLAB Function11/1(pr_actual_CP3), ChargingPoint3/1(powerRequest)  "pReq_CP3"
  ChargingPoint3/1(enablePowerFlow) -> Switch2/3, Switch2/2
  ElecritcVehicles3/2(plug) -> ChargingPoint3/2(plug)
  Delay6/1 -> MATLAB Function11/2(pr_previous_CP3)
  Product2/1 -> Switch2/1
  Delay8/1 -> ElecritcVehicles3/1(powerFlow)
  Power supply/1(y) -> Product2/1, Product1/1, Product/1
  Switch2/1 -> Delay8/1
  MATLAB Function4/1(y) -> Product2/2
  Delay7/1 -> MATLAB Function4/2(previous)
  Clock2/1 -> CP2/1(clock)
  Entity risposta4/1 -> Entity Replicator1/1
  Clock1/1 -> CP1/1(clock)
  Clock3/1 -> CP3/1(clock)
  Simulink Function2/1(Out1) -> Entity risposta5/1
  Entity Replicator4/3 -> Entity Multicast15/1
  Entity risposta5/1 -> Entity Replicator4/1
  Entity Replicator4/1 -> Entity Multicast4/1
  Entity Replicator4/2 -> Entity Multicast14/1
  Entity Replicator3/2 -> Entity Multicast13/1
  Entity risposta3/1 -> Entity Replicator3/1
  Entity Replicator3/1 -> Entity Multicast9/1
  Simulink Function6/1(Out1) -> Entity risposta3/1
  Entity Replicator5/1 -> Entity Multicast18/1
  Entity Replicator5/2 -> Entity Multicast16/1
  Entity Replicator5/3 -> Entity Multicast17/1
  Simulink Function8/1(Out1) -> Entity risposta6/1
  Entity risposta6/1 -> Entity Replicator5/1
  Entity risposta7/1 -> Entity Multicast19/1
  Simulink Function9/1(Out1) -> Entity risposta7/1
  MATLAB Function/1(y) -> Scope/1  "SOC_EV1"
  MATLAB Function1/1(y) -> Scope1/1  "SoC_EV2"
  MATLAB Function2/1(y) -> Scope2/1  "SoC_EV3"

== system CPS_PowerSync_System/ChargingPoint1/Error.Assignment ==
  powerRequest : Inport
  plug : Inport  Port=2
  Action Port : ActionPort
      settings: CopyFcn=Stateflow.SLINSF.SimulinkMan.removeBlockPreDeleteFcn  PreDeleteFcn=Stateflow.SLINSF.SimulinkMan.unsafePredeleteFcn
  Constant : Constant  Value=0  OutDataTypeStr=boolean
  enablePowerFlow : Outport
  wires:
  Constant/1 -> enablePowerFlow/1

== system CPS_PowerSync_System/ChargingPoint1/Normal.Connected.NotPowering.Assignment ==
  powerRequest : Inport
  plug : Inport  Port=2
  Action Port : ActionPort
      settings: CopyFcn=Stateflow.SLINSF.SimulinkMan.removeBlockPreDeleteFcn  PreDeleteFcn=Stateflow.SLINSF.SimulinkMan.unsafePredeleteFcn
  Constant : Constant  Value=0  OutDataTypeStr=boolean
  enablePowerFlow : Outport
  wires:
  Constant/1 -> enablePowerFlow/1

== system CPS_PowerSync_System/ChargingPoint1/Normal.Connected.Powering.Assignment ==
  powerRequest : Inport
  plug : Inport  Port=2
  Action Port : ActionPort
      settings: CopyFcn=Stateflow.SLINSF.SimulinkMan.removeBlockPreDeleteFcn  PreDeleteFcn=Stateflow.SLINSF.SimulinkMan.unsafePredeleteFcn
  Constant : Constant  OutDataTypeStr=boolean
  enablePowerFlow : Outport
  wires:
  Constant/1 -> enablePowerFlow/1

== system CPS_PowerSync_System/ChargingPoint1/Normal.Idle.Assignment ==
  powerRequest : Inport
  plug : Inport  Port=2
  Action Port : ActionPort
      settings: CopyFcn=Stateflow.SLINSF.SimulinkMan.removeBlockPreDeleteFcn  PreDeleteFcn=Stateflow.SLINSF.SimulinkMan.unsafePredeleteFcn
  Constant : Constant  Value=0  OutDataTypeStr=boolean
  enablePowerFlow : Outport
  wires:
  Constant/1 -> enablePowerFlow/1

== system CPS_PowerSync_System/ChargingPoint2/Error.Assignment ==
  powerRequest : Inport
  plug : Inport  Port=2
  Action Port : ActionPort
      settings: CopyFcn=Stateflow.SLINSF.SimulinkMan.removeBlockPreDeleteFcn  PreDeleteFcn=Stateflow.SLINSF.SimulinkMan.unsafePredeleteFcn
  Constant : Constant  Value=0  OutDataTypeStr=boolean
  enablePowerFlow : Outport
  wires:
  Constant/1 -> enablePowerFlow/1

== system CPS_PowerSync_System/ChargingPoint2/Normal.Connected.NotPowering.Assignment ==
  powerRequest : Inport
  plug : Inport  Port=2
  Action Port : ActionPort
      settings: CopyFcn=Stateflow.SLINSF.SimulinkMan.removeBlockPreDeleteFcn  PreDeleteFcn=Stateflow.SLINSF.SimulinkMan.unsafePredeleteFcn
  Constant : Constant  Value=0  OutDataTypeStr=boolean
  enablePowerFlow : Outport
  wires:
  Constant/1 -> enablePowerFlow/1

== system CPS_PowerSync_System/ChargingPoint2/Normal.Connected.Powering.Assignment ==
  powerRequest : Inport
  plug : Inport  Port=2
  Action Port : ActionPort
      settings: CopyFcn=Stateflow.SLINSF.SimulinkMan.removeBlockPreDeleteFcn  PreDeleteFcn=Stateflow.SLINSF.SimulinkMan.unsafePredeleteFcn
  Constant : Constant  OutDataTypeStr=boolean
  enablePowerFlow : Outport
  wires:
  Constant/1 -> enablePowerFlow/1

== system CPS_PowerSync_System/ChargingPoint2/Normal.Idle.Assignment ==
  powerRequest : Inport
  plug : Inport  Port=2
  Action Port : ActionPort
      settings: CopyFcn=Stateflow.SLINSF.SimulinkMan.removeBlockPreDeleteFcn  PreDeleteFcn=Stateflow.SLINSF.SimulinkMan.unsafePredeleteFcn
  Constant : Constant  Value=0  OutDataTypeStr=boolean
  enablePowerFlow : Outport
  wires:
  Constant/1 -> enablePowerFlow/1

== system CPS_PowerSync_System/ChargingPoint3/Error.Assignment ==
  powerRequest : Inport
  plug : Inport  Port=2
  Action Port : ActionPort
      settings: CopyFcn=Stateflow.SLINSF.SimulinkMan.removeBlockPreDeleteFcn  PreDeleteFcn=Stateflow.SLINSF.SimulinkMan.unsafePredeleteFcn
  Constant : Constant  Value=0  OutDataTypeStr=boolean
  enablePowerFlow : Outport
  wires:
  Constant/1 -> enablePowerFlow/1

== system CPS_PowerSync_System/ChargingPoint3/Normal.Connected.NotPowering.Assignment ==
  powerRequest : Inport
  plug : Inport  Port=2
  Action Port : ActionPort
      settings: CopyFcn=Stateflow.SLINSF.SimulinkMan.removeBlockPreDeleteFcn  PreDeleteFcn=Stateflow.SLINSF.SimulinkMan.unsafePredeleteFcn
  Constant : Constant  Value=0  OutDataTypeStr=boolean
  enablePowerFlow : Outport
  wires:
  Constant/1 -> enablePowerFlow/1

== system CPS_PowerSync_System/ChargingPoint3/Normal.Connected.Powering.Assignment ==
  powerRequest : Inport
  plug : Inport  Port=2
  Action Port : ActionPort
      settings: CopyFcn=Stateflow.SLINSF.SimulinkMan.removeBlockPreDeleteFcn  PreDeleteFcn=Stateflow.SLINSF.SimulinkMan.unsafePredeleteFcn
  Constant : Constant  OutDataTypeStr=boolean
  enablePowerFlow : Outport
  wires:
  Constant/1 -> enablePowerFlow/1

== system CPS_PowerSync_System/ChargingPoint3/Normal.Idle.Assignment ==
  powerRequest : Inport
  plug : Inport  Port=2
  Action Port : ActionPort
      settings: CopyFcn=Stateflow.SLINSF.SimulinkMan.removeBlockPreDeleteFcn  PreDeleteFcn=Stateflow.SLINSF.SimulinkMan.unsafePredeleteFcn
  Constant : Constant  Value=0  OutDataTypeStr=boolean
  enablePowerFlow : Outport
  wires:
  Constant/1 -> enablePowerFlow/1

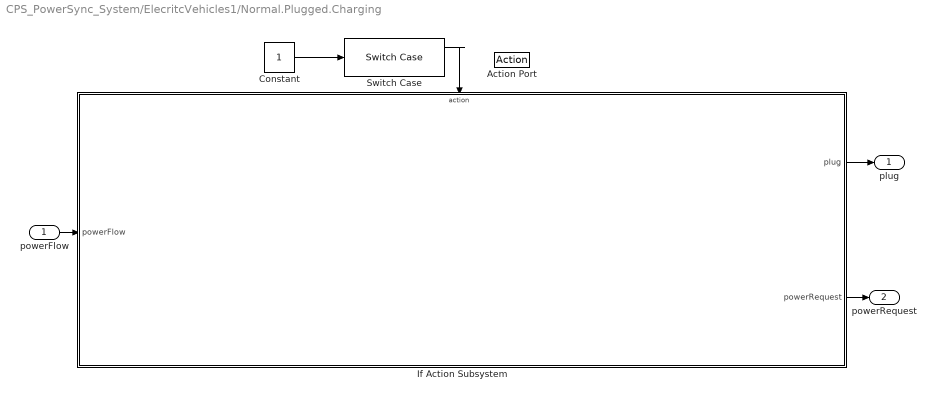
== system CPS_PowerSync_System/ElecritcVehicles1/Normal.Plugged.Charging ==
  powerFlow : Inport
  Action Port : ActionPort
      settings: CopyFcn=Stateflow.SLINSF.SimulinkMan.removeBlockPreDeleteFcn  PreDeleteFcn=Stateflow.SLINSF.SimulinkMan.unsafePredeleteFcn
  Constant : Constant
  If Action Subsystem : Subsystem  TreatAsAtomicUnit=on
  Switch Case : SwitchCase
  plug : Outport
  powerRequest : Outport  Port=2
  wires:
  powerFlow/1 -> If Action Subsystem/1(powerFlow)
  If Action Subsystem/1(plug) -> plug/1
  If Action Subsystem/2(powerRequest) -> powerRequest/1
  Constant/1 -> Switch Case/1
  Switch Case/1 -> If Action Subsystem/Action

== system CPS_PowerSync_System/ElecritcVehicles1/Normal.Plugged.Completed ==
  Action Port : ActionPort
      settings: CopyFcn=Stateflow.SLINSF.SimulinkMan.removeBlockPreDeleteFcn  PreDeleteFcn=Stateflow.SLINSF.SimulinkMan.unsafePredeleteFcn
  Constant : Constant
  If Action Subsystem : Subsystem  TreatAsAtomicUnit=on
  Switch Case : SwitchCase
  plug : Outport
  powerRequest : Outport  Port=2
  wires:
  Constant/1 -> Switch Case/1
  Switch Case/1 -> If Action Subsystem/Action
  If Action Subsystem/1(plug) -> plug/1
  If Action Subsystem/2(powerRequest) -> powerRequest/1

== system CPS_PowerSync_System/ElecritcVehicles1/Normal.Unplugged.Assigment ==
  powerFlow : Inport
  Action Port : ActionPort
      settings: CopyFcn=Stateflow.SLINSF.SimulinkMan.removeBlockPreDeleteFcn  PreDeleteFcn=Stateflow.SLINSF.SimulinkMan.unsafePredeleteFcn
  Constant : Constant  Value=0  OutDataTypeStr=boolean
  powerRequest : Outport
  plug : Outport  Port=2
  wires:
  Constant/1 -> powerRequest/1, plug/1

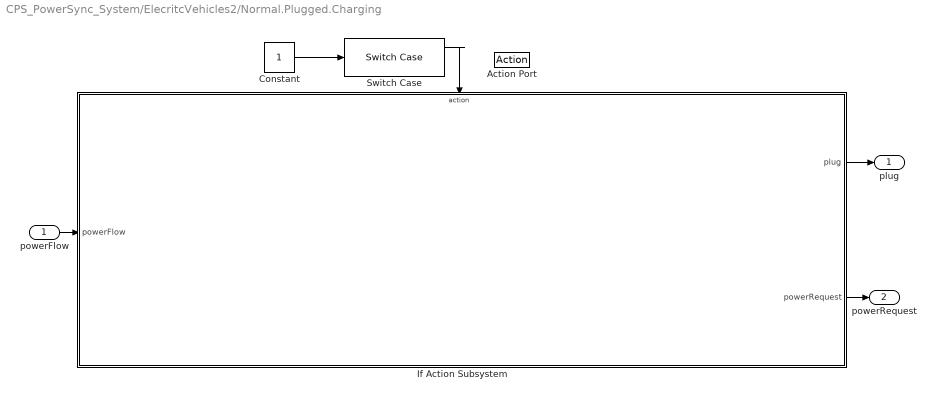
== system CPS_PowerSync_System/ElecritcVehicles2/Normal.Plugged.Charging ==
  powerFlow : Inport
  Action Port : ActionPort
      settings: CopyFcn=Stateflow.SLINSF.SimulinkMan.removeBlockPreDeleteFcn  PreDeleteFcn=Stateflow.SLINSF.SimulinkMan.unsafePredeleteFcn
  Constant : Constant
  If Action Subsystem : Subsystem  TreatAsAtomicUnit=on
  Switch Case : SwitchCase
  plug : Outport
  powerRequest : Outport  Port=2
  wires:
  Switch Case/1 -> If Action Subsystem/Action
  Constant/1 -> Switch Case/1
  If Action Subsystem/2(powerRequest) -> powerRequest/1
  If Action Subsystem/1(plug) -> plug/1
  powerFlow/1 -> If Action Subsystem/1(powerFlow)

== system CPS_PowerSync_System/ElecritcVehicles2/Normal.Plugged.Completed ==
  Action Port : ActionPort
      settings: CopyFcn=Stateflow.SLINSF.SimulinkMan.removeBlockPreDeleteFcn  PreDeleteFcn=Stateflow.SLINSF.SimulinkMan.unsafePredeleteFcn
  Constant : Constant
  If Action Subsystem : Subsystem  TreatAsAtomicUnit=on
  Switch Case : SwitchCase
  plug : Outport
  powerRequest : Outport  Port=2
  wires:
  If Action Subsystem/2(powerRequest) -> powerRequest/1
  If Action Subsystem/1(plug) -> plug/1
  Switch Case/1 -> If Action Subsystem/Action
  Constant/1 -> Switch Case/1

== system CPS_PowerSync_System/ElecritcVehicles2/Normal.Unplugged.Assigment ==
  powerFlow : Inport
  Action Port : ActionPort
      settings: CopyFcn=Stateflow.SLINSF.SimulinkMan.removeBlockPreDeleteFcn  PreDeleteFcn=Stateflow.SLINSF.SimulinkMan.unsafePredeleteFcn
  Constant : Constant  Value=0  OutDataTypeStr=boolean
  powerRequest : Outport
  plug : Outport  Port=2
  wires:
  Constant/1 -> plug/1, powerRequest/1

== system CPS_PowerSync_System/ElecritcVehicles3/Normal.Plugged.Charging ==
  powerFlow : Inport
  Action Port : ActionPort
      settings: CopyFcn=Stateflow.SLINSF.SimulinkMan.removeBlockPreDeleteFcn  PreDeleteFcn=Stateflow.SLINSF.SimulinkMan.unsafePredeleteFcn
  Constant : Constant
  If Action Subsystem : Subsystem  TreatAsAtomicUnit=on
  Switch Case : SwitchCase
  plug : Outport
  powerRequest : Outport  Port=2
  wires:
  powerFlow/1 -> If Action Subsystem/1(powerFlow)
  If Action Subsystem/1(plug) -> plug/1
  If Action Subsystem/2(powerRequest) -> powerRequest/1
  Constant/1 -> Switch Case/1
  Switch Case/1 -> If Action Subsystem/Action
